simulink model "schemat"  (R2020a)
settings: Solver=VariableStepAuto  StartTime=0.0  StopTime=10.0  RelTol=1e-3
values from neighbouring files (symbols this model uses):
  a = 4    [im.m]    (also in lab4ok.m)
  b = 13    [im.m]    (also in lab4ok.m)
  c = 3    [im.m]    (also in lab4ok.m)
  du = 0    [im.m]    (also in lab4ok.m = 1)
  k = 2    [im.m]    (also in lab4ok.m)
  u0 = 100    [im.m]    (also in lab4ok.m = 0)
  x0 = 0    [im.m]    (also in lab4ok.m)
  x10 = 0    [im.m]    (also in lab4ok.m)
settings Model: Creator=pc  LastModifiedBy=pc

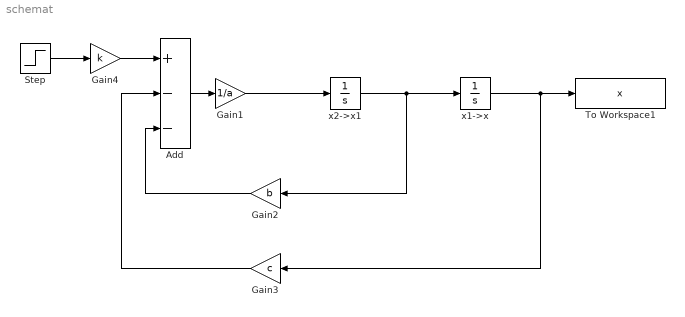
== system schemat ==
  Add : Sum  Inputs=+--
  Gain1 : Gain  Gain=1/a
  Gain2 : Gain  Gain=b
  Gain3 : Gain  Gain=c
  Gain4 : Gain  Gain=k
  Step : Step  Time=0  Before=u0  After=u0+du  SampleTime=1
  To Workspace1 : ToWorkspace  VariableName=x  SampleTime=-1
  x1->x : Integrator  InitialCondition=x0
  x2->x1 : Integrator  InitialCondition=x10
  wires:
  Step/1 -> Gain4/1
  Add/1 -> Gain1/1
  x2->x1/1 -> Gain2/1, x1->x/1
  Gain2/1 -> Add/3
  x1->x/1 -> Gain3/1, To Workspace1/1
  Gain3/1 -> Add/2
  Gain1/1 -> x2->x1/1
  Gain4/1 -> Add/1
